simulink model "simu_pid"  (R2018b)
settings: Solver=VariableStepAuto  StartTime=0.0  StopTime=5  RelTol=1e-3
values from neighbouring files (symbols this model uses):
  A = [                        0, 1, 0,                0 ... (first row only)    [sistema.m]
  B = [0; (-L*m*p1)/(M+m); 0; p2]    [sistema.m]
  C = eye(4)    [sistema.m]
  D = zeros(4,1)    [sistema.m]
  x0 = [0.2; 0; 0; 0]    [sistema.m]
undefined symbols (not defined in the file or in its folder): K
libraries: simulink x1
settings Model: Creator=vuvux  LastModifiedBy=vuvux

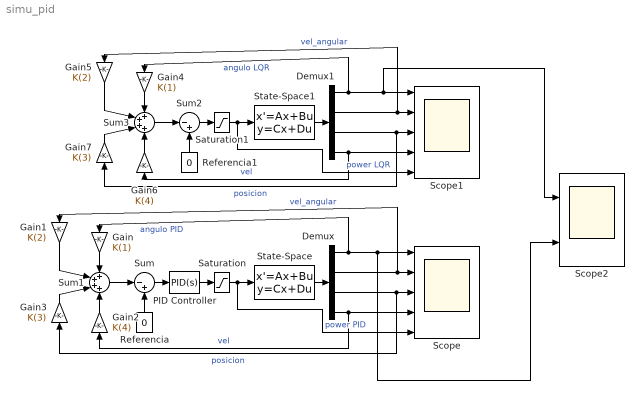
== system simu_pid ==
  Demux : Demux
  Demux1 : Demux
  Gain : Gain  Gain=K(1)
      settings: AttributesFormatString=%<Gain>
  Gain1 : Gain  Gain=K(2)
      settings: AttributesFormatString=%<Gain>
  Gain2 : Gain  Gain=K(4)
      settings: AttributesFormatString=%<Gain>
  Gain3 : Gain  Gain=K(3)
      settings: AttributesFormatString=%<Gain>
  Gain4 : Gain  Gain=K(1)
      settings: AttributesFormatString=%<Gain>
  Gain5 : Gain  Gain=K(2)
      settings: AttributesFormatString=%<Gain>
  Gain6 : Gain  Gain=K(4)
      settings: AttributesFormatString=%<Gain>
  Gain7 : Gain  Gain=K(3)
      settings: AttributesFormatString=%<Gain>
  PID Controller : simulink/Continuous/PID Controller  Controller=PID  Form=Parallel  TimeDomain=Continuous-time  SampleTime=-1  IntegratorMethod=Forward Euler  FilterMethod=Forward Euler  ControllerParametersSource=internal  P=2  I=3  D=0.01  UseFilter=on  N=100  TunerSelectOption=Transfer Function Based (PID Tuner App)  InitialConditionSource=internal  InitialConditionForIntegrator=0  InitialConditionForFilter=0  DifferentiatorICPrevScaledInput=0  ExternalReset=none  TrackingMode=off  Kt=1  LimitOutput=off  UpperSaturationLimit=inf  LowerSaturationLimit=-inf  LinearizeAsGain=on  AntiWindupMode=none  Kb=1  POutMin=[]  POutMax=[]  IOutMin=[]  IOutMax=[]  DOutMin=[]  DOutMax=[]  NOutMin=[]  NOutMax=[]  SumOutMin=[]  SumOutMax=[]  SaturationOutMin=[]  SaturationOutMax=[]  PParamMin=[]  PParamMax=[]  IParamMin=[]  IParamMax=[]  DParamMin=[]  DParamMax=[]  NParamMin=[]  NParamMax=[]  KbParamMin=[]  KbParamMax=[]  KtParamMin=[]  KtParamMax=[]  KbOutMin=[]  KbOutMax=[]  KtOutMin=[]  KtOutMax=[]  IntegratorOutMin=[]  IntegratorOutMax=[]  FilterOutMin=[]  FilterOutMax=[]  SumI1OutMin=[]  SumI1OutMax=[]  SumI2OutMin=[]  SumI2OutMax=[]  SumI3OutMin=[]  SumI3OutMax=[]  SumI4OutMin=[]  SumI4OutMax=[]  SumDOutMin=[]  SumDOutMax=[]  DifferentiatorOutMin=[]  DifferentiatorOutMax=[]  FilterDiffOutCoefMin=[]  FilterDiffOutCoefMax=[]  ReciprocalOutMin=[]  ReciprocalOutMax=[]  SumDenOutMin=[]  SumDenOutMax=[]  SumNumOutMin=[]  SumNumOutMax=[]  DivideOutMin=[]  DivideOutMax=[]  IntegratorContinuousStateAttributes=''  IntegratorStateMustResolveToSignalObject=off  IntegratorRTWStateStorageClass=Auto  FilterContinuousStateAttributes=''  FilterStateMustResolveToSignalObject=off  FilterRTWStateStorageClass=Auto  ParallelPVariant=InternalParameters  IdealPVariant=Disabled  IVariant=InternalParameters  DVariant=InternalParameters  IntegratorVariant=Continuous  SatVariant=Disabled  AWVariant=Passthrough  PCopyVariant=Disabled  TRVariant=Disabled  FdbkBlocksVariant=Forward  IdealPFdbkVariant=Disabled  SatFdbkVariant=Disabled  DerivativeFilterVariant=ContFilter  NVariant=InternalParameters  NCopyVariant=Disabled  FilterICVariant=InternalICsFilter  IntegratorICVariant=InternalICs  ExternalResetVariant=Disabled  TRSumVariant=Passthrough  SumFdbkVariant=Disabled  SumVariant=Sum_PID
  Referencia : Constant  Value=0
  Referencia1 : Constant  Value=0
  Saturation : Saturate  UpperLimit=5  LowerLimit=-5
  Saturation1 : Saturate  UpperLimit=5  LowerLimit=-5
  Scope : Scope  NumInputPorts=5
  Scope1 : Scope  NumInputPorts=5
  Scope2 : Scope  NumInputPorts=2
  State-Space : StateSpace  A=A  B=B  C=C  D=D  InitialCondition=x0
  State-Space1 : StateSpace  A=A  B=B  C=C  D=D  InitialCondition=x0
  Sum : Sum  Inputs=|-+
  Sum1 : Sum  Inputs=++++
  Sum2 : Sum  Inputs=|-+
  Sum3 : Sum  Inputs=++++
  wires:
  State-Space/1 -> Demux/1
  Demux/4 -> Scope/4, Gain2/1  "vel"
  Demux/1 -> Gain/1, Scope2/2, Scope/1  "angulo PID"
  Demux/2 -> Gain1/1, Scope/2  "vel_angular"
  Demux/3 -> Gain3/1, Scope/3  "posicion"
  Sum1/1 -> Sum/1
  Referencia/1 -> Sum/2
  Gain/1 -> Sum1/1
  Gain1/1 -> Sum1/2
  Gain2/1 -> Sum1/4
  Gain3/1 -> Sum1/3
  Saturation/1 -> Scope/5, State-Space/1  "power PID"
  PID Controller/1 -> Saturation/1
  Sum/1 -> PID Controller/1
  Referencia1/1 -> Sum2/2
  Demux1/1 -> Gain4/1, Scope2/1, Scope1/1  "angulo LQR"
  Saturation1/1 -> Scope1/5, State-Space1/1  "power LQR"
  Demux1/3 -> Gain7/1, Scope1/3  "posicion"
  Gain7/1 -> Sum3/3
  Demux1/4 -> Scope1/4, Gain6/1  "vel"
  State-Space1/1 -> Demux1/1
  Gain5/1 -> Sum3/2
  Sum3/1 -> Sum2/1
  Gain4/1 -> Sum3/1
  Sum2/1 -> Saturation1/1
  Gain6/1 -> Sum3/4
  Demux1/2 -> Gain5/1, Scope1/2  "vel_angular"
